simulink model "LKAS_AutoSave_DF_20220105_1052"  (R2018b)
settings: Solver=FixedStepDiscrete  StartTime=0.0  StopTime=10.0  FixedStep=0.01  RelTol=1e-3
InitFcn:
  | tmpVer = ver('MATLAB');
  | tmpVer = str2num(tmpVer.Version);
  | % -------------------------------------------------------------------
  | %  MATLAB file generated by Simulink.saveVars on 21-Nov-2019 10:06:14
  | %  MATLAB version: 7.13.0.564 (R2011b)
  | % -------------------------------------------------------------------
  | 
  | 
  | SInt16 = Simulink.AliasType;
  | SInt16.Description = 'Num';
  | if (tmpVer > 7.11)
  | 	SInt16.DataScope = 'Auto';
  | end
  | SInt16.HeaderFile = 'Rte_Type.h';
  | SInt16.BaseType = 'int16';
  | 
  | SInt32 = Simulink.AliasType;
  | SInt32.Description = 'Num';
  | if (tmpVer > 7.11)
  | 	SInt32.DataScope = 'Auto';
  | end
  | SInt32.HeaderFile = 'Rte_Type.h';
  | SInt32.BaseType = 'int32';
  | 
  | SInt8 = Simulink.AliasType;
  | SInt8.Description = 'Num';
  | if (tmpVer > 7.11)
  | 	SInt8.DataScope = 'Auto';
  | end
  | SInt8.HeaderFile = 'Rte_Type.h';
  | SInt8.BaseType = 'int8';
  | 
  | T_A_m2_1024_1_u32 = Simulink.NumericType;
  | T_A_m2_1024_1_u32.Description = 'm2 (square meters  (m2))';
  | if (tmpVer > 7.11)
  | 	T_A_m2_1024_1_u32.DataScope = 'Auto';
  | end
  | T_A_m2_1024_1_u32.HeaderFile = 'Rte_Type.h';
  | T_A_m2_1024_1_u32.DataTypeMode = 'Fixed-point: slope and bias scaling';
  | T_A_m2_1024_1_u32.SignednessBool = false;
  | T_A_m2_1024_1_u32.WordLength = 32;
  | T_A_m2_1024_1_u32.FixedExponent = -10;
  | T_A_m2_1024_1_u32.SlopeAdjustmentFactor = 1;
  | T_A_m2_1024_1_u32.Bias = 0;
  | T_A_m2_1024_1_u32.DataTypeOverride = 'Inherit';
  | T_A_m2_1024_1_u32.IsAlias = true;
  | 
  | T_A_m2_65536_1_u16 = Simulink.NumericType;
  | T_A_m2_65536_1_u16.Description = 'm2 (square meters  (m2))';
  | if (tmpVer > 7.11)
  | 	T_A_m2_65536_1_u16.DataScope = 'Auto';
  | end
  | T_A_m2_65536_1_u16.HeaderFile = 'Rte_Type.h';
  | T_A_m2_65536_1_u16.DataTypeMode = 'Fixed-point: slope and bias scaling';
  | T_A_m2_65536_1_u16.SignednessBool = false;
  | T_A_m2_65536_1_u16.WordLength = 16;
  | T_A_m2_65536_1_u16.FixedExponent = -16;
  | T_A_m2_65536_1_u16.SlopeAdjustmentFactor = 1;
  | T_A_m2_65536_1_u16.Bias = 0;
  | T_A_m2_65536_1_u16.DataTypeOverride = 'Inherit';
  | ... (+4647 lines)
StopFcn:
  | clear  T_A_m2_1024_1_u32 T_A_m2_65536_1_u16 T_A_m2_Float32 T_A_mm2_10_1_u16 T_A_mm2_4_1_s16 T_A_mm2_Float32 T_Cnt_Num_10_1_u32 T_Cnt_Num_1_1_s16 T_Cnt_Num_1_1_s32 T_Cnt_Num_1_1_s8 T_Cnt_Num_1_1_u16 T_Cnt_Num_1_1_u32 T_Cnt_Num_1_1_u8 T_E_J_1_1_s32 T_E_J_Float32 T_E_kJ_128_1_s32 T_E_kJ_Float32 T_E_kwh_10_1_u16 T_E_kwh_Float32 T_Epl_kwhpkm_100_1_u16 T_Epl_kwhpkm_Float32 T_F_N_1_1_s16 T_F_N_Float32 T_I_A_1000_1_u16 T_I_A_1048576_1_s32 T_I_A_2048_1_s16 T_I_A_32_1_s16 T_I_A_Float32 T_I_mA_1_1_s16 T_I_mA_32768_128_s16 T_I_mA_Float32 T_J_kgpm2_128_1_u16 T_J_kgpm2_Float32 T_K_NA_1000_1_s16 T_K_NA_100_1_s16 T_K_NA_100_1_u16 T_K_NA_1024_1_s16 T_K_NA_1024_1_u16 T_K_NA_128_1_s16 T_K_NA_128_1_u16 T_K_NA_128_1_u8 T_K_NA_16777216_1_u32 T_K_NA_16_1_s16 T_K_NA_16_1_u16 T_K_NA_16_1_u8 T_K_NA_1_16_u16 T_K_NA_1_1_s16 T_K_NA_1_1_u16 T_K_NA_1_1_u8 T_K_NA_32768_1_s16 T_K_NA_32768_1_u16 T_K_NA_32_1_s8 T_K_NA_4096_1_u16 T_K_NA_4194304_1_s32 T_K_NA_4194304_1_u16 T_K_NA_65536_1_s32 T_K_NA_65536_1_u16 T_K_NA_8192_1_s16 T_K_NA_8_1_s16 T_K_NA_Float32 T_M_Nm_16_1_s16 T_M_Nm_1_1_s16 T_M_Nm_32768_1_s16 T_M_Nm_32_1_s16 T_M_Nm_4_1_s16 T_M_Nm_512_1_s16 T_M_Nm_Float32 T_P_W_1_4_s16 T_P_W_1_8_s16 T_P_W_Float32 T_P_kW_128_1_s16 T_P_kW_1_8_s16 T_P_kW_8_1_s32 T_P_kW_Float32 T_Pct_pct_1024_1_s32 T_Pct_pct_1024_1_u32 T_Pct_pct_10_1_s16 T_Pct_pct_10_1_u32 T_Pct_pct_128_100_s8 T_Pct_pct_1_1_s16 T_Pct_pct_1_4_u8 T_Pct_pct_255_100_u16 T_Pct_pct_255_100_u8 T_Pct_pct_256_1_s16 T_Pct_pct_256_1_u16 T_Pct_pct_65535_100_u16 T_Pct_pct_Float32 T_R_ohm_1024_1_s16 T_R_ohm_32_1_s16 T_R_ohm_Float32 T_TK_K_16_1_s16 T_TK_K_Float32 T_T_degC_10_400_1_u16 T_T_degC_16_1_s16 T_T_degC_1_40_1_u8 T_T_degC_2_80_1_u8 T_T_degC_Float32 T_U_V_1000_1_u16 T_U_V_10_1_u8 T_U_V_200_1_u8 T_U_V_32_1_s16 T_U_V_4096_1_s16 T_U_V_512_1_s16 T_U_V_65535_8_u16 T_U_V_8192_1_u16 T_U_V_Float32 T_U_mV_1_1_s16 T_U_mV_256_20_u16 T_U_mV_Float32 T_V_l_256_1_s16 T_V_l_4096_1_s16 T_V_l_64_1_s16 T_V_l_65535_100_u16 T_V_l_Float32 T_V_ml_128_1_s16 T_V_ml_1_1_s16 T_V_ml_32768_1_s16 T_V_ml_Float32 T_V_ul_32_1_u16 T_V_ul_Float32 T_Vpl_clpkm_512_1_u16 T_Vpl_clpkm_Float32 T_a_kphps_16_1_s16 T_a_kphps_Float32 T_a_mps2_128_1_s16 T_a_mps2_Float32 T_c_MJpkg_256_1_s16 T_c_MJpkg_Float32 T_c_kJpgpK_1024_1_s16 T_c_kJpgpK_Float32 T_c_kJpkgpK_128_1_u16 T_c_kJpkgpK_Float32 T_chrg_Ah_1_1_s16 T_chrg_Ah_1_1_u16 T_chrg_Ah_1_1_u8 T_chrg_Ah_256_1_u16 T_chrg_Ah_4194304_1_s32 T_chrg_Ah_512_1_u16 T_chrg_Ah_8_1_u16 T_chrg_Ah_Float32 T_cmp_NA_100_1_s16 T_cmp_NA_128_1_s16 T_cmp_NA_16_1_s16 T_cmp_NA_32768_1_u16 T_cmp_NA_Float32 T_d2n_rpmps2_4_1_s16 T_d2n_rpmps2_Float32 T_dPct_pctps_16_1_s16 T_dPct_pctps_256_1_s16 T_dPct_pctps_Float32 T_dT_degCps_128_1_s16 T_dT_degCps_Float32 T_dV_lph_1_1_s16 T_dV_lph_Float32 T_dV_lpm_128_1_s16 T_dV_lpm_32_1_s16 T_dV_lpm_Float32 T_dV_lps_1024_1_u16 T_dV_lps_4_1_u16 T_dV_lps_Float32 T_dV_mlps_1024_1_s16 T_dV_mlps_Float32 T_d_BitField16 T_dm_gps_128_1_s16 T_dm_gps_128_1_u16 T_dm_gps_256_1_u16 T_dm_gps_Float32 T_dm_mgps_1_1_s16 T_dm_mgps_Float32 T_dn_rpmps_1_1_s16 T_dn_rpmps_2_1_s16 T_dn_rpmps_Float32 T_dp_Paps_1_1_s16 T_dp_Paps_Float32 T_dp_kPaps_1_1_s16 T_dp_kPaps_8_1_s16 T_dp_kPaps_Float32 T_dphi_degps_128_1_s16 T_dphi_degps_8_1_s16 T_dphi_degps_Float32 T_dr_ps_256_1_s16 T_dr_ps_Float32 T_drho_mgplps_1_2_s16 T_drho_mgplps_Float32 T_e_NA_1_1_u8 T_f_Hz_1_1_u16 T_f_Hz_1_1_u32 T_f_Hz_64_1_u16 T_f_Hz_8_1_s16 T_f_Hz_Float32 T_g_BitField32 T_l_km_16_1_s16 T_l_km_1_1_u16 T_l_km_1_1_u32 T_l_km_Float32 T_l_m_1024_1_s16 T_l_m_16_1_s16 T_l_m_1_1_u32 T_l_m_Float32 T_l_mm_16_1_s16 T_l_mm_1_1_u16 T_l_mm_4096_1_s16 T_l_mm_4_1_u8 T_l_mm_64_1_s16 T_l_mm_Float32 T_m_g_1_1_s16 T_m_g_2048_1_s16 T_m_g_32_1_u16 T_m_g_Float32 T_m_kg_1024_1_s16 T_m_kg_1_1_s16 T_m_kg_1_1_u32 T_m_kg_Float32 T_m_mg_128_1_s16 T_m_mg_32_1_s16 T_m_mg_Float32 T_n_rpm_1_1_s16 T_n_rpm_1_25_u8 T_n_rpm_256_50_u16 T_n_rpm_2_25_u8 T_n_rpm_4_1_u16 T_n_rpm_Float32 T_p_MPa_64_1_s16 T_p_MPa_Float32 T_p_Pa_1_1_s16 T_p_Pa_Float32 T_p_kPa_1_10_u16 T_p_kPa_1_1_s16 T_p_kPa_1_1_u8 T_p_kPa_256_1_u16 T_p_kPa_32_1_u16 T_p_kPa_64_1_s16 T_p_kPa_Float32 T_phi_deg_100_1_s16 T_phi_deg_1024_1_s16 T_phi_deg_128_1_s16 T_phi_deg_1_1_u8 T_phi_deg_256_1_s16 T_phi_deg_2_1_s8 T_phi_deg_32_1_s16 T_phi_deg_512_6_s32 T_phi_deg_Float32 T_phi_rad_2048_1_s16 T_phi_rad_Float32 T_r_NA_1024_1_s16 T_r_NA_1024_1_u16 T_r_NA_16384_1_s16 T_r_NA_16_1_s16 T_r_NA_256_1_s8 T_r_NA_256_1_u16 T_r_NA_32768_1_u16 T_r_NA_32_1_u16 T_r_NA_4096_1_s16 T_r_NA_65535_2_u16 T_r_NA_8192_1_u16 T_r_NA_Float32 T_rho_gpl_8192_1_s16 T_rho_gpl_Float32 T_rho_kgpm3_16_1_s16 T_rho_kgpm3_Float32 T_rho_mgpl_1_1_s16 T_rho_mgpl_64_1_s16 T_rho_mgpl_Float32 T_t_hour_1_1_s16 T_t_hour_Float32 T_t_m_1_1_u16 T_t_m_Float32 T_t_ms_1_1_s16 T_t_ms_1_1_u16 T_t_ms_1_1_u32 T_t_ms_4096_1_s16 T_t_ms_64_1_s16 T_t_ms_Float32 T_t_s_1000_1_s16 T_t_s_100_1_s16 T_t_s_10_1_s16 T_t_s_10_1_u16 T_t_s_1_1_s16 T_t_s_1_1_u16 T_t_s_1_1_u32 T_t_s_Float32 T_t_us_10_1_u32 T_t_us_1_1_s16 T_t_us_1_1_u32 T_t_us_1_4_u16 T_t_us_Float32 T_v_kph_1_1_u8 T_v_kph_64_1_s16 T_v_kph_64_1_u16 T_v_kph_Float32 T_v_mps_256_1_s16 T_v_mps_Float32 T_w_radps_32_1_s16 T_w_radps_Float32 T_y_BitField8 T_y_BitFieldDiagProgress T_y_BitFieldDiagStatus T_y_NA_1_1_u8 SInt16 SInt32 SInt8 T_BOOLEAN UInt16 UInt32 UInt8 s16 s32 s8 u16 u32 u8
model workspace (MAT data in the model file):
  MCOS : class17 (value not decoded)
  MCOS : class17 (value not decoded)
  MCOS : class17 (value not decoded)
  MCOS : class17 (value not decoded)
  MCOS : class17 (value not decoded)
  MCOS : class17 (value not decoded)
  MCOS : class17 (value not decoded)
  MCOS : class17 (value not decoded)
  MCOS : class17 (value not decoded)
  MCOS : class17 (value not decoded)
  MCOS : class17 (value not decoded)
  MCOS : class17 (value not decoded)
  MCOS : class17 (value not decoded)
  MCOS : class17 (value not decoded)
  MCOS : class17 (value not decoded)
  MCOS : class17 (value not decoded)
  MCOS : class17 (value not decoded)
  MCOS : class17 (value not decoded)
  MCOS : class17 (value not decoded)
  MCOS : class17 (value not decoded)
  MCOS : class17 (value not decoded)
  MCOS : class17 (value not decoded)
  MCOS : class17 (value not decoded)
  MCOS : class17 (value not decoded)
  MCOS : class17 (value not decoded)
  MCOS : class17 (value not decoded)
  MCOS : class17 (value not decoded)
  MCOS : class17 (value not decoded)
  MCOS : class17 (value not decoded)
  MCOS : class17 (value not decoded)
  MCOS : class17 (value not decoded)
  MCOS : class17 (value not decoded)
  MCOS : class17 (value not decoded)
  MCOS : class17 (value not decoded)
  MCOS : class17 (value not decoded)
  MCOS : class17 (value not decoded)
  MCOS : class17 (value not decoded)
  MCOS : class17 (value not decoded)
  MCOS : class17 (value not decoded)
  MCOS : class17 (value not decoded)
  MCOS : class17 (value not decoded)
  MCOS : class17 (value not decoded)
  MCOS : class17 (value not decoded)
  MCOS : class17 (value not decoded)
  MCOS : class17 (value not decoded)
  MCOS : class17 (value not decoded)
  MCOS : class17 (value not decoded)
  MCOS : class17 (value not decoded)
  MCOS : class17 (value not decoded)
  MCOS : class17 (value not decoded)
  MCOS : class17 (value not decoded)
  MCOS : class17 (value not decoded)
  MCOS : class17 (value not decoded)
  MCOS : class17 (value not decoded)
  MCOS : class17 (value not decoded)
  MCOS : class17 (value not decoded)
  MCOS : class17 (value not decoded)
  MCOS : class17 (value not decoded)
  MCOS : class17 (value not decoded)
  MCOS : class17 (value not decoded)
  MCOS : class17 (value not decoded)
  MCOS : class17 (value not decoded)
  MCOS : class17 (value not decoded)
  MCOS : class17 (value not decoded)
  MCOS : class17 (value not decoded)
  MCOS : class17 (value not decoded)
  MCOS : class17 (value not decoded)
  MCOS : class17 (value not decoded)
  MCOS : class17 (value not decoded)
  MCOS : class17 (value not decoded)
  MCOS : class17 (value not decoded)
  MCOS : class17 (value not decoded)
  MCOS : class17 (value not decoded)
  MCOS : class17 (value not decoded)
  MCOS : class17 (value not decoded)
  MCOS : class17 (value not decoded)
  MCOS : class17 (value not decoded)
  MCOS : class17 (value not decoded)
  MCOS : class17 (value not decoded)
  MCOS : class17 (value not decoded)
  MCOS : class17 (value not decoded)
  MCOS : class17 (value not decoded)
  MCOS : class17 (value not decoded)
  MCOS : class17 (value not decoded)
  MCOS : class17 (value not decoded)
  MCOS : class17 (value not decoded)
  MCOS : class17 (value not decoded)
  MCOS : class17 (value not decoded)
  MCOS : class17 (value not decoded)
  MCOS : class17 (value not decoded)
  MCOS : class17 (value not decoded)
  MCOS : class17 (value not decoded)
  MCOS : class17 (value not decoded)
  MCOS : class17 (value not decoded)
  MCOS : class17 (value not decoded)
  MCOS : class17 (value not decoded)
  MCOS : class17 (value not decoded)
undefined symbols (not defined in the file): LKA_CarWidth, LKA_SampleTime, LKA_StrRatio_C, LKA_Veh2CamL_C, LKA_Veh2CamW_C, LKA_WhlBaseL_C, LL_CompSWA_C, LL_CrvtPrvwT_C, LL_DesDvt_C, LL_DvtComp_C, LL_DvtPrvwT_C, LL_DvtSpdDet_vDvtSpdMin_C, LL_HdAgExT_C, LL_HdAgPrvwT_C, LL_LAccMax_C, LL_LAccRMax_C, LL_LDW_EarliestWarnLine_C, LL_LDW_LatestWarnLine_C, LL_LDWS_SUPPRESS_HEADING, LL_LFClb_TFC_FfCtlRatio_C, LL_LFClb_TFC_KdBalance_C, LL_LFClb_TFC_KdMaxSWA_C, LL_LFClb_TFC_KdV1_C, LL_LFClb_TFC_KdV2_C, LL_LFClb_TFC_KdVehSpdLwr_C, LL_LFClb_TFC_KdVehSpdUpr_C, LL_LFClb_TFC_Ki_C, LL_LFClb_TFC_KiMaxSWA_C, LL_LFClb_TFC_Kp_C, LL_LFClb_TFC_KpKlat_C, LL_LFClb_TFC_KpV1_C, LL_LFClb_TFC_KpV2_C, LL_LFClb_TFC_KpVehSpdLwr_C, LL_LFClb_TFC_KpVehSpdUpr_C, LL_LFClb_TFC_PrvwT_C, LL_LKA_EarliestWarnLine_C, LL_LKA_LatestWarnLine_C, LL_LKAExPrcs_ExitC0Dvt, LL_LKAExPrcs_ExitC0Swt, LL_LKAExPrcs_tiExitTime1, LL_LKAExPrcs_tiExitTime2, LL_LKAExPrcs_tiExitTime3, LL_LKAS_OUT_OF_CONTROL_LAT_VEL, LL_LKAS_OUT_OF_CONTROL_TTLC, LL_LKASWASyn_M0, LL_LKASWASyn_M1, LL_LKASWASyn_M2, LL_LKASWASyn_M3K, LL_LKASWASyn_SWAaddMax, LL_LKASWASyn_T2, LL_LKASWASyn_tiTrqSwaRtTime, LL_LKASWASyn_tiTrqSwaTime, LL_LKASWASyn_TrqMax, LL_LKASWASyn_TrqSwaAddSwt, LL_LKASWASyn_TrqSwaRateDiff, LL_LSpdCompT_C, LL_lStpLngth_C, LL_MAX_DELAY_EPSSTAR_TIME, LL_MAX_DRIVER_TORQUE_DISABLE, LL_MAX_DRIVER_TORQUE_ENABLE ... (+38)
libraries: simulink x138, canmsglib x8, dspstat3 x3, simulink_extras x1
(part 19 of 19)

== matlab function LKAS_AutoSave_DF_20220105_1052/LKAS/LL/LLOn/LKA/LKA Motion Planning (LKAMP) /Steering Wheel Angle Command Calculation (SWACmdCal)/SWACmd ==
  data: SWACmd_dphi1PhSWAGrad input; SWACmd_phi2PhSWAIni input; SWACmd_dphi2PhSWAGrad input; SWACmd_phi1PhSWAIni input; SWACmd_phiSWACmd output single; SWACmd_tiNomT input; T1 output single; T2 output
 function [SWACmd_phiSWACmd,T1,T2] = SWACmd(SWACmd_dphi1PhSWAGrad,...
                                                      SWACmd_phi2PhSWAIni,...
                                                      SWACmd_dphi2PhSWAGrad,...
                                                      SWACmd_phi1PhSWAIni,...
                                                      SWACmd_tiNomT)                      
% *************************************************************************
% 输入量：
%   SWACmd_phi1PhSWAIni : 一区转向盘转角初始值，单位：deg
%   SWACmd_dphi1PhSWAGrad : 一区转向盘转角变化率，单位：deg/s
%   SWACmd_phi2PhSWAIni : 二区转向盘转角初始值，单位：deg
%   SWACmd_dphi2PhSWAGrad : 二区转向盘转角变化率，单位：deg/s
%   SWACmd_vVehSpdIni : 进入一区的车速初始值，单位：Km/h
%   SWACmd_tiNomT : 名义时间，单位：s
%
% 输出量：
%   SWACmd_phiSWACmd : 转向盘转角指令值，单位：deg
%  
%**************************************************************************
%
    DelteSW0 = SWACmd_phi1PhSWAIni; 
    DelteSW1 = SWACmd_phi2PhSWAIni;
    Delte1PhSWGrad = SWACmd_dphi1PhSWAGrad;
    Delte2PhSWGrad = SWACmd_dphi2PhSWAGrad;
    DelteSWCmd = single(0);
    NomT = SWACmd_tiNomT;
    T1 = (DelteSW1-DelteSW0)/Delte1PhSWGrad;
    T2 = (0-DelteSW1)/Delte2PhSWGrad+T1;
%**************************************************************************
%已知： 一区转向盘转角初始值， 一区转向盘转角变化率， 二区转向盘转角初始值, 
%       二区转向盘转角变化率, 进入一区的车速初始值, 行驶路径长度。
%根据车速初始值和行驶路径长度，可以计算出名义时间（NomT）；然后利用名义时间和
%方向盘运动曲线，求得转向盘转角指令值。
%
%**************************************************************************                                
if(NomT < T1 && NomT >= 0 )
    DelteSWCmd = DelteSW0+Delte1PhSWGrad*NomT;
elseif(NomT <= T2 && NomT >= T1 )
%    DelteSWCmd = DelteSW1+Delte2PhSWGrad*(NomT-T1);
    DelteSWCmd = DelteSW0+Delte1PhSWGrad*T1;
%    DelteSWCmd = single(0);
elseif(NomT >= T2)
    DelteSWCmd = DelteSW0+Delte1PhSWGrad*T1;
%   DelteSWCmd = single(0);
end
%
%**************************************************************************
% 输出：
    SWACmd_phiSWACmd = DelteSWCmd;
end

== matlab function LKAS_AutoSave_DF_20220105_1052/LKAS/LL/LLOn/LKA/Lane Following (LF)/Trajectory Following Control (TFC)/Feedback Control (FbCtl)/Saturable Gain Lut (SatGainLut) ==
  data: Input input single [0..180]; Gain output single [10..400]; InputLimLwr input single; InputLimUpr input single; GainLimLwr input single; GainLimUpr input single
%% Function Name: Saturable Gain Lut
%
% Description: 
%   Saturable Gain Lookup Table.
%
% Assumptions and Limitation:
%   The data type of all inputs and output is single.
%
% Inputs:
%   Input:
%   InputLimLwr:
%   InputLimUpr:
%   GainLimLwr:
%   GainLimUpr:
%
% Outputs:
%   Gain: The result of Looking up table.

% $Revision: 1.0$
% $Author: Zhang Jianwei$
% $Date: January 27, 2019$
% ________________________________________
function Gain = fcn(Input, InputLimLwr, InputLimUpr, GainLimLwr, GainLimUpr)
%#eml
if Input <= InputLimLwr
    Gain = GainLimLwr;
elseif Input >= InputLimUpr
        Gain = GainLimUpr;
else Gain = (Input - InputLimLwr)/(InputLimUpr - InputLimLwr)...
        *(GainLimUpr - GainLimLwr) + GainLimLwr;
end
end

== matlab function LKAS_AutoSave_DF_20220105_1052/LKAS/LL/LLOn/LKA/Lane Following (LF)/Trajectory Following Control (TFC)/Feedback Control (FbCtl)/Saturable Gain Lut (SatGainLut)1 ==
  data: Input input single [0..180]; Gain output single [10..400]; InputLimLwr input single; InputLimUpr input single; GainLimLwr input single; GainLimUpr input single
%% Function Name: Saturable Gain Lut
%
% Description: 
%   Saturable Gain Lookup Table.
%
% Assumptions and Limitation:
%   The data type of all inputs and output is single.
%
% Inputs:
%   Input:
%   InputLimLwr:
%   InputLimUpr:
%   GainLimLwr:
%   GainLimUpr:
%
% Outputs:
%   Gain: The result of Looking up table.

% $Revision: 1.0$
% $Author: Zhang Jianwei$
% $Date: January 27, 2019$
% ________________________________________
function Gain = fcn(Input, InputLimLwr, InputLimUpr, GainLimLwr, GainLimUpr)
%#eml
if Input <= InputLimLwr
    Gain = GainLimLwr;
elseif Input >= InputLimUpr
        Gain = GainLimUpr;
else Gain = (Input - InputLimLwr)/(InputLimUpr - InputLimLwr)...
        *(GainLimUpr - GainLimLwr) + GainLimLwr;
end
end

== matlab function LKAS_AutoSave_DF_20220105_1052/LKAS/LL/LLOn/LKA Input Processing (LKAInP)/TTLC Calculation (TTLCCalc)/MATLAB Function ==
  data: dvt input; vy input; TTLC output; cur input
function TTLC = fcn(dvt, vy, cur)
    if dvt>single(0) && dvt<single(2) && vy<single(0) && vy>single(-1.5)
        TTLC = -dvt/vy;
    else
        TTLC = single(3);
    end
end

== matlab function LKAS_AutoSave_DF_20220105_1052/LKAS/LL/LLOn/LKA Input Processing (LKAInP)/TTLC Calculation (TTLCCalc)/MATLAB Function1 ==
  data: dvt input; vy input; TTLC output; cur input
function TTLC = fcn(dvt, vy, cur)
    if dvt>single(0) && dvt<single(2) && vy<single(0) && vy>single(-1.5)
        TTLC = (-dvt)/vy;
    else
        TTLC = single(3);
    end
end

== matlab function LKAS_AutoSave_DF_20220105_1052/LKAS/LL/LLOn/LKA Input Processing (LKAInP)/TTLC Calculation (TTLCCalc)/MATLAB Function2 ==
  data: crPrvwCrvtLft input; crPrvwCrvtRgt input; LTLC input; RTLC input; LFTTTLC output; LTTLC input; RTTLC input; RGTTTLC output; TLft input; TRgt input
function [LFTTTLC,RGTTTLC] = fcn(crPrvwCrvtLft, crPrvwCrvtRgt, LTLC, RTLC, LTTLC, RTTLC ,TLft, TRgt)
    if abs(LTTLC-LTLC)/LTTLC <= single(0.2)
        LFTTTLC = min(LTTLC,LTLC);
    else
        LFTTTLC = LTTLC;
    end
    
    if abs(RTTLC-RTLC)/RTTLC <= single(0.2)
        RGTTTLC = min(RTTLC,RTLC);
    else
        RGTTTLC = RTTLC;
    end
    
    if abs(crPrvwCrvtLft)>single(0.001) && abs(TLft-LFTTTLC)/LFTTTLC <= single(0.7) && TLft>single(0.5) && LFTTTLC <= single(1.95)
        LFTTTLC = (LFTTTLC+TLft)/single(2);
    end
    if abs(crPrvwCrvtRgt)>single(0.001) && abs(TRgt-RGTTTLC)/RGTTTLC <= single(0.7) && TRgt>single(0.5) && RGTTTLC <= single(1.95)
        RGTTTLC = (RGTTTLC+TRgt)/single(2);
    end
end

== matlab function LKAS_AutoSave_DF_20220105_1052/LKAS/LL/LLOn/LKA Input Processing (LKAInP)/TTLC Calculation (TTLCCalc)/MATLAB Function3 ==
  data: c0 input; TLft output; c1 input; c2 input; vx input; c20 input; w input
function TLft = fcn(c0,c1,c2,vx,c20,w)
%   y1=c0+c1*x+c2*x^2+c3*x^3
%   y2=-W + C20*x^2
%   y1-y2 =(c2-c20)*x^2+c1*x+(c0+w)=0
%   b2-4ac=c1^2-4*(c2-c20)*(c0+w)
    if (c2-c20)<=single(0.001) && ((c1 > 0) || (c1 < 0))
        if (-c0-w)/c1>0
            TLft = (-c0-w)/c1/vx;
        else
            TLft = single(3);
        end
    elseif ((c2-c20)>single(0.001)) && (c1^2-4*(c2-c20)*(c0+w) >= 0)
        x10= (-c1+sqrt(c1^2-4*(c2-c20)*(c0+w)))/(2*(c2-c20));
        x20= (-c1-sqrt(c1^2-4*(c2-c20)*(c0+w)))/(2*(c2-c20));
        x1 = max(x10,x20);
        x2 = min(x10,x20);
        if x2>0
            TLft = x2/vx;
        elseif x1>0
            TLft = x1/vx;
        else
            TLft = single(3);
        end
    else
        TLft = single(3);
    end
    TLft =max(single(0.6),min(TLft,single(2)));
end

== matlab function LKAS_AutoSave_DF_20220105_1052/LKAS/LL/LLOn/LKA Input Processing (LKAInP)/TTLC Calculation (TTLCCalc)/MATLAB Function4 ==
  data: c0 input; TRgt output; c1 input; c2 input; vx input; c20 input; w input
function TRgt = fcn(c0,c1,c2,vx,c20,w)
%   y1=c0+c1*x+c2*x^2+c3*x^3
%   y2=W + C20*x^2
%   y1-y2 =(c2-c20)*x^2+c1*x+(c0-w)=0
%   b2-4ac=c1^2-4*(c2-c20)*(c0-w)
    if (c2-c20)<=single(0.001) && ((c1 > 0) || (c1 < 0))
        if (-c0+w)/c1>0
            TRgt = (-c0+w)/c1/vx;
        else
            TRgt = single(3);
        end
    elseif ((c2-c20)>single(0.001)) && (c1^2-4*(c2-c20)*(c0-w) >= 0)
        x10= (-c1+sqrt(c1^2-4*(c2-c20)*(c0-w)))/(2*(c2-c20));
        x20= (-c1-sqrt(c1^2-4*(c2-c20)*(c0-w)))/(2*(c2-c20));
        x1 = max(x10,x20);
        x2 = min(x10,x20);
        if x2>0
            TRgt = x2/vx;
        elseif x1>0
            TRgt = x1/vx;
        else
            TRgt = single(3);
        end
    else
        TRgt = single(3);
    end
    TRgt =max(single(0.6),min(TRgt,single(2)));
end

== matlab function LKAS_AutoSave_DF_20220105_1052/LKAS/LL/LLOn/LKA Input Processing (LKAInP)/TTLC Calculation (TTLCCalc)/MATLAB Function5 ==
  data: vx input; sw_angle input; TTLC output; WhlBaseL_C input; StrRatio_C input
function TTLC = fcn(vx,sw_angle,WhlBaseL_C,StrRatio_C)
   K = 0.09/vx;
   TTLC = sw_angle/((1+K*vx*vx)*WhlBaseL_C*StrRatio_C*2);
end

== matlab function LKAS_AutoSave_DF_20220105_1052/LKAS/LL/LLOn/LKA Input Processing (LKAInP)/Under The Limit (UndrLim)/Steering Wheel Angel Max (SWAMax)/MATLAB Function ==
  data: v input; SWAmax output; ax input; i input; L input; K input
function SWAmax = get_SWAmax(v,ax,i,L,K)
SWAmax = ((K*v*v+1)*ax*i*L)/(v*v)*180/3.14;

== matlab function LKAS_AutoSave_DF_20220105_1052/LKAS/LL/LLOn/LKA Input Processing (LKAInP)/Under The Limit (UndrLim)/Steering Wheel Angel Rate Max (SWARMax)/MATLAB Function ==
  data: v input; SWARmax output; dax input; i input; L input; K input
function SWARmax = get_SWARmax(v,dax,i,L,K)
SWARmax = ((K*v*v+1)*dax*i*L)/(v*v)*180/3.14;

== stateflow chart LKAS_AutoSave_DF_20220105_1052/LKAS/LL/LLOn/LL State Determination (LLStateDet)/LDW_State_Machine ==
  state SysOn
    state LDWSelected
      en:
      LDWSM_stLDWState = uint16(2);
    state Normal
      state LDWEnable
        en:
        LDWSM_stLDWState = uint16(3);
      state LDWLeftActive
        en:
        LDWSM_stLDWState = uint16(4);
        LDWSM_stLDWActvFlg = uint16(1);
        ex:
        LDWSM_stLDWActvFlg = uint16(0);
      state LDWRightActive
        en:
        LDWSM_stLDWState = uint16(5);
        LDWSM_stLDWActvFlg = uint16(2);
        ex:
        LDWSM_stLDWActvFlg = uint16(0);
      (default) -> LDWEnable
      LDWEnable -> LDWRightActive [order 2] : [LDWSM_stActvCSyn == 2 & LDWSM_stDeactvCSyn == 0]
      LDWEnable -> LDWLeftActive [order 1] : [LDWSM_stActvCSyn == 1 & LDWSM_stDeactvCSyn == 0]
      LDWLeftActive -> LDWEnable [order 1] : [LDWSM_stDeactvCSyn == 1]
      LDWRightActive -> LDWEnable [order 1] : [LDWSM_stDeactvCSyn == 1]
      LDWLeftActive -> LDWRightActive [order 2] : [LDWSM_stActvCSyn == 2 & LDWSM_stDeactvCSyn == 0]
      LDWRightActive -> LDWLeftActive [order 2] : [LDWSM_stActvCSyn == 1 & LDWSM_stDeactvCSyn == 0]
    (default) -> LDWSelected
    LDWSelected -> Normal : [LDWSM_stEnaCSyn == 1&LDWSM_stDisblCSyn==0]
    Normal -> LDWSelected : [LDWSM_stDisblCSyn == 1]
  state SysOff
    state Unavailable
      en:
      LDWSM_stLDWState = uint16(0);
    state Unselected
      en:
      LDWSM_stLDWState = uint16(1);
    (default) -> Unavailable
    Unavailable -> Unselected : [LDWSM_stLMCMode == 0]
  state Fault
    state LDWFault
      en:
      LDWSM_stLDWState = uint16(6);
    (default) -> LDWFault
  (default) -> SysOff
  SysOff -> SysOn [order 2] : [LDWSM_stLMCMode == 1 | LDWSM_stLMCMode == 2]
  SysOn -> Unselected [order 2] : [LDWSM_stLMCMode ~= 1 & LDWSM_stLMCMode ~= 2 ]
  Fault -> Unselected [order 2] : [LDWSM_stLMCMode == 0 & LDWSM_stFaultCSyn == 0]
  SysOff -> Fault [order 1] : [(LDWSM_stLMCMode == 1 | LDWSM_stLMCMode == 2) & LDWSM_stFaultCSyn == 1]
  SysOn -> Fault [order 1] : [LDWSM_stFaultCSyn == 1]
  Fault -> SysOn [order 1] : [LDWSM_stFaultCSyn == 0 & (LDWSM_stLMCMode == 1 | LDWSM_stLMCMode == 2) ]
  data: LDWSM_stLDWActvFlg output uint8 [0..7]; LDWSM_stLDWState output uint8 [0..7]; LDWSM_stLMCMode input uint8 [0..5]; LDWSM_stEnaCSyn input boolean [0..1]; LDWSM_stDisblCSyn input boolean [0..1]; LDWSM_stActvCSyn input uint8 [0..3]; LDWSM_stDeactvCSyn input boolean [0..1]; LDWSM_stFaultCSyn input boolean [0..1]
  data LDWSM_stLDWActvFlg settings: description=|
      | 0 -- Deactive
      | 1 -- Left Active
      | 2 -- Right Active
  data LDWSM_stLDWState settings: description=|
      | 0 -- Unavailable
      | 1 -- Unselected
      | 2 -- Selected
      | 3 -- Enabled
      | 4 -- Left Active
      | 5 -- Right Active
      | 6 -- Fault
      | 7 -- Reserved
  data LDWSM_stLMCMode settings: description=|
      | 0 -- Unselected
      | 1 -- LDWMode
      | 2 -- LKAMode
      | 3 -- TJAMode
      | 4 -- HWAMode
      | 5 -- Reserved
  data LDWSM_stEnaCSyn settings: description=|
      | 0 -- No Enable
      | 1 -- LDW Enable
      | 2 -- LKA Enable
      | 3 -- Reserved
  data LDWSM_stDisblCSyn settings: description=|
      | 0 -- No Disable
      | 1 -- LDW Disable
      | 2 -- LKA Disable
      | 3 -- Reserved
  data LDWSM_stActvCSyn settings: description=|
      | 0 -- No Active
      | 1 -- LDW Left Active
      | 2 -- LDW Right Active
      | 3 -- LKA Left Active
      | 4 -- LKA Right Active
      | 5 -- Reserved
  data LDWSM_stDeactvCSyn settings: description=|
      | 0 -- No Deactive
      | 1 -- LDW Deactive
      | 2 -- LKA Deactive
      | 3 -- Reserved
  data LDWSM_stFaultCSyn settings: description=|
      | 0 -- No Fault
      | 1 -- LDW Fault
      | 2 -- LKA Fault
      | 3 -- Reserved

== stateflow chart LKAS_AutoSave_DF_20220105_1052/LKAS/LL/LLOn/LL State Determination (LLStateDet)/LKA_State_Machine ==
  state SysOn
    state LKASelected
      en:
      LKASM_stLKAState = uint16(2);
    state Normal
      state LKAEnable
        en:
        LKASM_stLKAState = uint16(3);
      state LKALeftActive
        en:
        LKASM_stLKAState = uint16(4);
        LKASM_stLKAActvFlg = uint16(1);
        ex:
        LKASM_stLKAActvFlg = uint16(0);
      state LKARightActive
        en:
        LKASM_stLKAState = uint16(5);
        LKASM_stLKAActvFlg = uint16(2);
        ex:
        LKASM_stLKAActvFlg = uint16(0);
      (default) -> LKAEnable
      LKAEnable -> LKARightActive [order 2] : [LKASM_stActvCSyn == 2 & LKASM_stDeactvCSyn ==0 ]
      LKAEnable -> LKALeftActive [order 1] : [LKASM_stActvCSyn == 1 & LKASM_stDeactvCSyn ==0 ]
      LKALeftActive -> LKAEnable [order 1] : [LKASM_stDeactvCSyn ==1 ]
      LKARightActive -> LKAEnable [order 1] : [LKASM_stDeactvCSyn == 1]
      LKALeftActive -> LKARightActive [order 2] : [LKASM_stActvCSyn == 2 & LKASM_stDeactvCSyn ==0]
      LKARightActive -> LKALeftActive [order 2] : [LKASM_stActvCSyn == 1 & LKASM_stDeactvCSyn ==0]
    (default) -> LKASelected
    LKASelected -> Normal : [LKASM_stEnaCSyn == 1&LKASM_stDisblCSyn ==0]
    Normal -> LKASelected : [LKASM_stDisblCSyn ==1]
  state SysOff
    state Unavailable
      en:
      LKASM_stLKAState = uint16(0);
    state Unselected
      en:
      LKASM_stLKAState = uint16(1);
    (default) -> Unavailable
    Unavailable -> Unselected : [LKASM_stLMCMode == 0 | LKASM_stLMCMode == 1]
  state Fault
    state LKAFault
      en:
      LKASM_stLKAState = uint16(6);
    (default) -> LKAFault
  (default) -> SysOff
  SysOff -> SysOn [order 2] : [LKASM_stLMCMode == 2]
  SysOn -> Unselected [order 2] : [LKASM_stLMCMode ~= 2]
  Fault -> Unselected [order 2] : [(LKASM_stLMCMode == 0 | LKASM_stLMCMode == 1) & LKASM_stFaultCSyn == 0]
  SysOff -> Fault [order 1] : [LKASM_stLMCMode == 2 & LKASM_stFaultCSyn == 1 ]
  SysOn -> Fault [order 1] : [LKASM_stFaultCSyn == 1 ]
  Fault -> SysOn [order 1] : [LKASM_stFaultCSyn == 0 & LKASM_stLMCMode == 2]
  data: LKASM_stLKAActvFlg output uint8 [0..7]; LKASM_stLKAState output uint8 [0..7]; LKASM_stLMCMode input uint8 [0..5]; LKASM_stEnaCSyn input boolean [0..1]; LKASM_stDisblCSyn input boolean [0..1]; LKASM_stActvCSyn input uint8 [0..3]; LKASM_stDeactvCSyn input boolean [0..1]; LKASM_stFaultCSyn input boolean [0..1]
  data LKASM_stLKAActvFlg settings: description=|
      | 0 -- Deactive
      | 1 -- Left Active
      | 2 -- Right Active
  data LKASM_stLKAState settings: description=|
      | 0 -- Unavailable
      | 1 -- Unselected
      | 2 -- Selected
      | 3 -- Enabled
      | 4 -- Left Active
      | 5 -- Right Active
      | 6 -- Fault
      | 7 -- Reserved
  data LKASM_stLMCMode settings: description=|
      | 0 -- Unselected
      | 1 -- LDWMode
      | 2 -- LKAMode
      | 3 -- TJAMode
      | 4 -- HWAMode
      | 5 -- Reserved
  data LKASM_stEnaCSyn settings: description=|
      | 0 -- No Enable
      | 1 -- LDW Enable
      | 2 -- LKA Enable
      | 3 -- Reserved
  data LKASM_stDisblCSyn settings: description=|
      | 0 -- No Disable
      | 1 -- LDW Disable
      | 2 -- LKA Disable
      | 3 -- Reserved
  data LKASM_stActvCSyn settings: description=|
      | 0 -- No Active
      | 1 -- LDW Left Active
      | 2 -- LDW Right Active
      | 3 -- LKA Left Active
      | 4 -- LKA Right Active
      | 5 -- Reserved
  data LKASM_stDeactvCSyn settings: description=|
      | 0 -- No Deactive
      | 1 -- LDW Deactive
      | 2 -- LKA Deactive
      | 3 -- Reserved
  data LKASM_stFaultCSyn settings: description=|
      | 0 -- No Fault
      | 1 -- LDW Fault
      | 2 -- LKA Fault
      | 3 -- Reserved

== matlab function LKAS_AutoSave_DF_20220105_1052/LKAS/LL/LLOn/LL State Determination (LLStateDet)/LL State Machine Conditions (LLSMCon)/Activation Condition (ActvC)/Deviation Threshold Condition (DvtThresCon)/Active Lane Calculation (ActLanCalc)/MATLAB Function ==
  data: LaneWidth input; ThresDet_coefficient output; LKA_CarWidth input; DvtThresUprLDW input
function ThresDet_coefficient = fcn(LaneWidth, LKA_CarWidth, DvtThresUprLDW)
   LanWidmin = single(LKA_CarWidth+single(2)*DvtThresUprLDW);
   LanWidmax = single(LKA_CarWidth+single(6)*DvtThresUprLDW);

    LanWid = single(min(max(LanWidmin,LaneWidth), LanWidmax));
    k = single(LanWid-single(LKA_CarWidth+single(single(2)*DvtThresUprLDW)))/single(4*DvtThresUprLDW);
    ThresDet_coefficient = single(min(max(single(0),k),single(1)));
end

== matlab function LKAS_AutoSave_DF_20220105_1052/LKAS/LL/LLOn/LL State Determination (LLStateDet)/LL State Machine Conditions (LLSMCon)/Deactivation Condition (DeactvC)/Deviation Threshold Condition (DvtThresCon)/Active Lane Calculation (ActLanCalc)/MATLAB Function ==
  data: LaneWidth input; ThresDet_coefficient output; LKA_CarWidth input; DvtThresUprLDW input
function ThresDet_coefficient = fcn(LaneWidth, LKA_CarWidth, DvtThresUprLDW)
    LanWidmin = single(LKA_CarWidth+single(2)*DvtThresUprLDW);
    LanWidmax = single(LKA_CarWidth+single(6)*DvtThresUprLDW);
    LanWid = single(min(max(LanWidmin,LaneWidth), LanWidmax));
    k = single(LanWid-single(LKA_CarWidth+single(single(2)*DvtThresUprLDW)))/single(4*DvtThresUprLDW);
    ThresDet_coefficient = single(min(max(single(0),k),single(1)));
end

== matlab function LKAS_AutoSave_DF_20220105_1052/LKAS/LL/LLOn/LL State Determination (LLStateDet)/LL State Machine Conditions (LLSMCon)/Deactivation Condition (DeactvC)/Driver Take Condition (DvrTkCon)/MATLAB Function ==
  data: stActvFlg input; stDvrTkConFlg output; EPSTrq input; VehSpd input; DisableTrq input; PrvwCrvt input
function stDvrTkConFlg = fcn(stActvFlg, EPSTrq, VehSpd, DisableTrq,PrvwCrvt)
    Spd = single(min(max(single(60),VehSpd),single(80)));
    Crvt = single(min(max(single(-0.005),PrvwCrvt),single(0.005)));
    CrvtTrq = (abs(Crvt))/single(0.005);
    MidTqlmt = single((single(1.5)*DisableTrq-Spd/single(120)*DisableTrq)*single(0.8) + CrvtTrq);
    if stActvFlg == 2 && EPSTrq > MidTqlmt
        stDvrTkConFlg=1;
    elseif stActvFlg == 1 && EPSTrq < single(-1)*MidTqlmt
        stDvrTkConFlg=1;
    else
        stDvrTkConFlg=0;
    end
end

== matlab function LKAS_AutoSave_DF_20220105_1052/LKAS/LL/LLOn/LL State Determination (LLStateDet)/LL State Machine Conditions (LLSMCon)/Disable Condition (DisblC)/Driver Intent Condition (DrvInttC)/Take-Over Steering Check (TkOvStChk)/MATLAB Function ==
  data: VehSpd input; stDvrTkConFlg output; EPSTrq input; DisableTrq input; PrvwCrvt input
function stDvrTkConFlg = fcn(VehSpd,EPSTrq,DisableTrq,PrvwCrvt)
    CrvtTrq = single(abs(PrvwCrvt)/single(0.005));
    MidTqlmt = single(single(1.5)*DisableTrq-VehSpd/single(180)*DisableTrq + CrvtTrq);
    Tqlmt = single(min(max(single(1.5),MidTqlmt),single(2.75)));
    if EPSTrq >= Tqlmt
        stDvrTkConFlg=true;
    else
        stDvrTkConFlg=false;
    end
end

== matlab function LKAS_AutoSave_DF_20220105_1052/LKAS/LL/LLOn/LL State Determination (LLStateDet)/LL State Machine Conditions (LLSMCon)/Disable Condition (DisblC)/Subsystem/C1 ==
  data: u input; y output
function y = fcn(u)
if u==0

  y=1;
else
    y=0;
end

== matlab function LKAS_AutoSave_DF_20220105_1052/LKAS/LL/LLOn/LL State Determination (LLStateDet)/LL State Machine Conditions (LLSMCon)/Disable Condition (DisblC)/Subsystem/CURVAT ==
  data: u input; y output
function y = fcn(u)
if u==0

  y=1;
else
    y=0;
end

== matlab function LKAS_AutoSave_DF_20220105_1052/LKAS/LL/LLOn/LL State Determination (LLStateDet)/LL State Machine Conditions (LLSMCon)/Disable Condition (DisblC)/Subsystem/GEAR ==
  data: u input; y output
function y = fcn(u)
if u==0

  y=1;
else
    y=0;
end

== matlab function LKAS_AutoSave_DF_20220105_1052/LKAS/LL/LLOn/LL State Determination (LLStateDet)/LL State Machine Conditions (LLSMCon)/Disable Condition (DisblC)/Subsystem/LDWOwn ==
  data: u input; y output
function y = fcn(u)
if u==0

  y=1;
else
    y=0;
end

== matlab function LKAS_AutoSave_DF_20220105_1052/LKAS/LL/LLOn/LL State Determination (LLStateDet)/LL State Machine Conditions (LLSMCon)/Disable Condition (DisblC)/Subsystem/LDWTimeOut ==
  data: u input; y output
function y = fcn(u)
if u==0

  y=1;
else
    y=0;
end

== matlab function LKAS_AutoSave_DF_20220105_1052/LKAS/LL/LLOn/LL State Determination (LLStateDet)/LL State Machine Conditions (LLSMCon)/Disable Condition (DisblC)/Subsystem/LIGHT ==
  data: u input; y output
function y = fcn(u)
if u==0

  y=1;
else
    y=0;
end

== matlab function LKAS_AutoSave_DF_20220105_1052/LKAS/LL/LLOn/LL State Determination (LLStateDet)/LL State Machine Conditions (LLSMCon)/Disable Condition (DisblC)/Subsystem/LKA_EPS ==
  data: u input; y output
function y = fcn(u)
if u==0

  y=1;
else
    y=0;
end

== matlab function LKAS_AutoSave_DF_20220105_1052/LKAS/LL/LLOn/LL State Determination (LLStateDet)/LL State Machine Conditions (LLSMCon)/Disable Condition (DisblC)/Subsystem/LKA_LATSPEED ==
  data: u input; y output
function y = fcn(u)
if u==0

  y=1;
else
    y=0;
end

== matlab function LKAS_AutoSave_DF_20220105_1052/LKAS/LL/LLOn/LL State Determination (LLStateDet)/LL State Machine Conditions (LLSMCon)/Disable Condition (DisblC)/Subsystem/LKA_POS ==
  data: u input; y output
function y = fcn(u)
if u==0

  y=1;
else
    y=0;
end

== matlab function LKAS_AutoSave_DF_20220105_1052/LKAS/LL/LLOn/LL State Determination (LLStateDet)/LL State Machine Conditions (LLSMCon)/Disable Condition (DisblC)/Subsystem/Q ==
  data: u input; y output
function y = fcn(u)
if u==0

  y=1;
else
    y=0;
end

== matlab function LKAS_AutoSave_DF_20220105_1052/LKAS/LL/LLOn/LL State Determination (LLStateDet)/LL State Machine Conditions (LLSMCon)/Disable Condition (DisblC)/Subsystem/RELEASE ==
  data: u input; y output
function y = fcn(u)
if u==0

  y=1;
else
    y=0;
end

== matlab function LKAS_AutoSave_DF_20220105_1052/LKAS/LL/LLOn/LL State Determination (LLStateDet)/LL State Machine Conditions (LLSMCon)/Disable Condition (DisblC)/Subsystem/SPEED ==
  data: u input; y output
function y = fcn(u)
if u==0

  y=1;
else
    y=0;
end

== matlab function LKAS_AutoSave_DF_20220105_1052/LKAS/LL/LLOn/LL State Determination (LLStateDet)/LL State Machine Conditions (LLSMCon)/Disable Condition (DisblC)/Subsystem/SWA ==
  data: u input; y output
function y = fcn(u)
if u==0

  y=1;
else
    y=0;
end

== matlab function LKAS_AutoSave_DF_20220105_1052/LKAS/LL/LLOn/LL State Determination (LLStateDet)/LL State Machine Conditions (LLSMCon)/Disable Condition (DisblC)/Subsystem/SWARate ==
  data: u input; y output
function y = fcn(u)
if u==0

  y=1;
else
    y=0;
end

== matlab function LKAS_AutoSave_DF_20220105_1052/LKAS/LL/LLOn/LL State Determination (LLStateDet)/LL State Machine Conditions (LLSMCon)/Disable Condition (DisblC)/Subsystem/Takeover ==
  data: u input; y output
function y = fcn(u)
if u==0

  y=1;
else
    y=0;
end

== matlab function LKAS_AutoSave_DF_20220105_1052/LKAS/LL/LLOn/LL State Determination (LLStateDet)/LL State Machine Conditions (LLSMCon)/Disable Condition (DisblC)/Subsystem/WIDTH ==
  data: u input; y output
function y = fcn(u)
if u==0

  y=1;
else
    y=0;
end

== matlab function LKAS_AutoSave_DF_20220105_1052/LKAS/LL/LLOn/LL State Determination (LLStateDet)/LL State Machine Conditions (LLSMCon)/Disable Condition (DisblC)/Subsystem/aFLAcc ==
  data: u input; y output
function y = fcn(u)
if u==0

  y=1;
else
    y=0;
end

== matlab function LKAS_AutoSave_DF_20220105_1052/LKAS/LL/LLOn/LL State Determination (LLStateDet)/LL State Machine Conditions (LLSMCon)/Disable Condition (DisblC)/Subsystem/aLAcc ==
  data: u input; y output
function y = fcn(u)
if u==0

  y=1;
else
    y=0;
end

== matlab function LKAS_AutoSave_DF_20220105_1052/LKAS/LL/LLOn/LL State Determination (LLStateDet)/LL State Machine Conditions (LLSMCon)/Disable Condition (DisblC)/Subsystem1/Disable Reason ==
  data: u input; y output
function y = DisableReason(u)
y = single(0);
 for i = 1:18
    if u(i) == 1
        y = single(i);
        break
    end
 end
end

== matlab function LKAS_AutoSave_DF_20220105_1052/LKAS/LL/LLOn/LL State Determination (LLStateDet)/LL State Machine Conditions (LLSMCon)/Enable Condition (EnaC)/LDW Own Condition (LDWOwnC)/Vehicle Position Check (VehPosChk)/Subsystem/MATLAB Function ==
  data: DvtThresUprLDW input; LaneWidth input; ThresDet_coefficient output; LKA_CarWidth input
function ThresDet_coefficient = fcn(DvtThresUprLDW,LaneWidth, LKA_CarWidth)
   LanWidmin = single(LKA_CarWidth+single(2)*DvtThresUprLDW);
   LanWidmax = single(LKA_CarWidth+single(6)*DvtThresUprLDW);
   LanWid = single(min(max(LanWidmin,LaneWidth), LanWidmax));
    k = single(LanWid-single(LKA_CarWidth+single(single(2)*DvtThresUprLDW)))/single(4*DvtThresUprLDW);
    ThresDet_coefficient = single(min(max(single(0),k),single(1)));
end

== matlab function LKAS_AutoSave_DF_20220105_1052/LKAS/LL/LLOn/LL State Determination (LLStateDet)/LL State Machine Conditions (LLSMCon)/Enable Condition (EnaC)/LKA Own Condition (LKAOwnC)/Vehicle Position Check (VehPosChk)1/Subsystem/MATLAB Function ==
  data: DvtThresUprLDW input; LaneWidth input; ThresDet_coefficient output; LKA_CarWidth input
function ThresDet_coefficient = fcn(DvtThresUprLDW,LaneWidth, LKA_CarWidth)
   LanWidmin = single(LKA_CarWidth+single(2)*DvtThresUprLDW);
   LanWidmax = single(LKA_CarWidth+single(6)*DvtThresUprLDW);
   LanWid = single(min(max(LanWidmin,LaneWidth), LanWidmax));
    k = single(LanWid-single(LKA_CarWidth+single(single(2)*DvtThresUprLDW)))/single(4*DvtThresUprLDW);
    ThresDet_coefficient = single(min(max(single(0),k),single(1)));
end
